simulink model "lab1_simulink"  (R2021a)
settings: Solver=VariableStepAuto  StartTime=0.0  StopTime=8  RelTol=1e-3
model workspace (MAT data in the model file):
  K_ss = 0.0433
values from neighbouring files (symbols this model uses):
  J_tot = 7.226    [lab1_script.m]    (also in lab1_simulink_script.m)
  k_b = 2    [lab1_script.m]    (also in lab1_simulink_script.m)
  K_cs = 0.5    [lab1_script.m]    (also in lab1_simulink_script.m)
  k_f = 0.1    [lab1_script.m]    (also in lab1_simulink_script.m)
  m_tot__K_t = 1.8    [lab1_script.m]    (also in lab1_simulink_script.m)
  p_Cw_A_vo_r__i_tot = 0.6154    [lab1_script.m]    (also in lab1_simulink_script.m)
  r__i_tot = 0.0615    [lab1_script.m]    (also in lab1_simulink_script.m)
  R_a = 1    [lab1_script.m]    (also in lab1_simulink_script.m)
libraries: simulink x4
settings Model: EnablePacing=on  Creator=Ahmed  LastModifiedBy=Ahmed

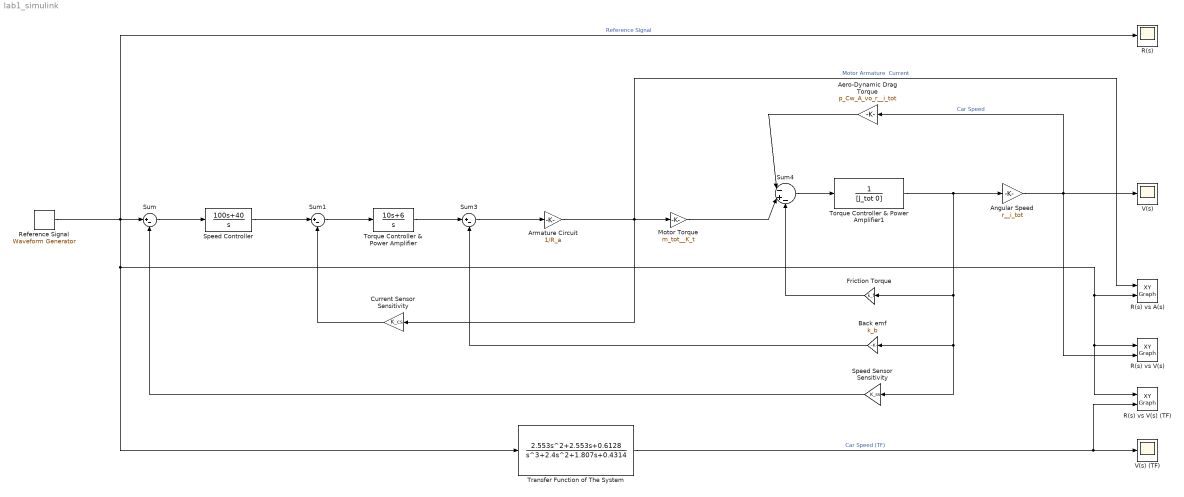
== system lab1_simulink ==
  Aero-Dynamic Drag Torque : Gain  Gain=p_Cw_A_vo_r__i_tot
  Angular Speed : Gain  Gain=r__i_tot
  Armature Circuit : Gain  Gain=1/R_a
  Back emf : Gain  Gain=k_b
  Current Sensor Sensitivity : Gain  Gain=K_cs
  Friction Torque : Gain  Gain=k_f
  Motor Torque : Gain  Gain=m_tot__K_t
  R(s) : Scope
  R(s) vs A(s) : simulink/Sinks/XY Graph  xmin=-6  xmax=6  ymin=-10  ymax=10  st=-1
  R(s) vs V(s) : simulink/Sinks/XY Graph  xmin=-1  xmax=1  ymin=-1  ymax=1  st=-1
  R(s) vs V(s) (TF) : simulink/Sinks/XY Graph  xmin=-1  xmax=1  ymin=-1  ymax=1  st=-1
  Reference Signal : simulink/Sources/Waveform Generator  OutMin=[]  OutMax=[]  OutDataTypeStr=double  SelectedSignal=2  Signals=step('StepTime',0,'InitialValue',0,'FinalValue',2)#sin('Amplitude',2,'Frequency',300,'Phase',0)#sawtooth('Amplitude',5,'Frequency',1)#square('Amplitude',1,'Frequency',10,'Phase',0,'DutyCycle',50)#pulse('Amplitude',1,'TriggerTime',1,'Duration',2)#step('StepTime',1,'InitialValue',0,'FinalValue',4)#sin('Amplitude',4,'Frequency',200,'Phase',pi/2)#sawtooth('Amplitude',2.5,'Frequency',10)#square('Amplitude',5,'Frequency',5,'Phase',0,'DutyCycle',80)#pulse('Amplitude',4,'TriggerTime',2,'Duration',5)  BlockNames=MultiportSwitch_c9a01619ac3f4f5#MultiportSwitch_627b212c998e4cf#MultiportSwitch_8229cf88104f40d#MultiportSwitch_c1ad6828debd43b#MultiportSwitch_13722959f0df4c2#MultiportSwitch_9298adaa41c942c#MultiportSwitch_2be25b026c5447d#MultiportSwitch_5c1ef7ebcdb441d#MultiportSwitch_87e6ded30da4430#MultiportSwitch_61e886d4a9c5407  SampleTime=0.5
  Speed Controller : TransferFcn  Numerator=[100 40]  Denominator=[1 0]
  Speed Sensor Sensitivity : Gain  Gain=K_ss
  Sum : Sum  Inputs=|+-
  Sum1 : Sum  Inputs=|+-
  Sum3 : Sum  Inputs=|+-
  Sum4 : Sum  Inputs=|-+-
  Torque Controller & Power Amplifier : TransferFcn  Numerator=[10 6]  Denominator=[1 0]
  Torque Controller & Power Amplifier1 : TransferFcn  Numerator=[0 1]  Denominator=[J_tot 0]
  Transfer Function of The System : TransferFcn  Numerator=[0 2.553 2.553 0.6128]  Denominator=[1 2.4 1.807 0.4314]
  V(s) : Scope
  V(s) (TF) : Scope
  wires:
  Reference Signal/1 -> R(s)/1, Transfer Function of The System/1, R(s) vs A(s)/2, R(s) vs V(s) (TF)/1, R(s) vs V(s)/1, Sum/1  "Reference Signal"
  Sum/1 -> Speed Controller/1
  Speed Sensor Sensitivity/1 -> Sum/2
  Speed Controller/1 -> Sum1/1
  Sum1/1 -> Torque Controller & Power Amplifier/1
  Torque Controller & Power Amplifier/1 -> Sum3/1
  Sum3/1 -> Armature Circuit/1
  Armature Circuit/1 -> R(s) vs A(s)/1, Current Sensor Sensitivity/1, Motor Torque/1  "Motor Armature  Current"
  Motor Torque/1 -> Sum4/2
  Sum4/1 -> Torque Controller & Power Amplifier1/1
  Friction Torque/1 -> Sum4/3
  Torque Controller & Power Amplifier1/1 -> Angular Speed/1, Speed Sensor Sensitivity/1, Back emf/1, Friction Torque/1
  Aero-Dynamic Drag Torque/1 -> Sum4/1
  Angular Speed/1 -> R(s) vs V(s)/2, V(s)/1, Aero-Dynamic Drag Torque/1  "Car Speed"
  Back emf/1 -> Sum3/2
  Current Sensor Sensitivity/1 -> Sum1/2
  Transfer Function of The System/1 -> R(s) vs V(s) (TF)/2, V(s) (TF)/1  "Car Speed (TF)"
